simulink model "gm_TapFilter"  (R2017a)
settings: Solver=VariableStepAuto  StartTime=0.0  StopTime=10.0  RelTol=1e-3
settings Model: Creator=Arthur  LastModifiedBy=Arthur
settings OptimizationCC: BlockReduction=off  ConditionallyExecuteInputs=off
settings DebuggingCC: InheritedTsInSrcMsg=none

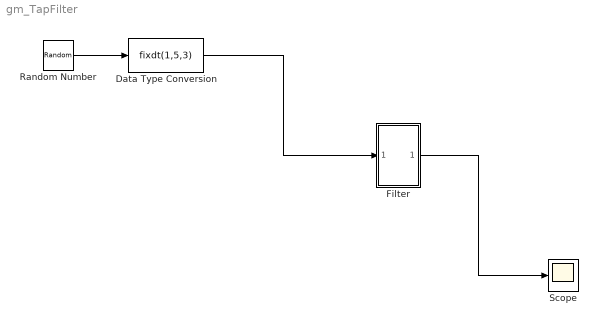
== system gm_TapFilter ==
  Data Type Conversion : DataTypeConversion  OutDataTypeStr=fixdt(1,5,3)
  Filter : Subsystem
  Random Number : RandomNumber  SampleTime=0.1
  Scope : Scope
  wires:
  Filter/1(Out1) -> Scope/1
  Data Type Conversion/1 -> Filter/1(In1)
  Random Number/1 -> Data Type Conversion/1

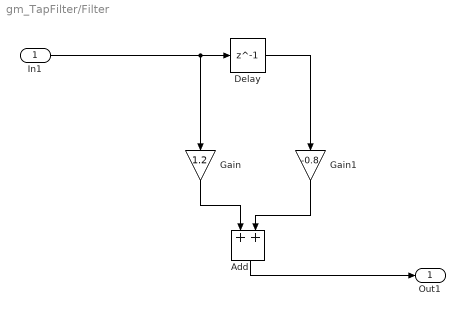
== system gm_TapFilter/Filter ==
  In1 : Inport
  Add : Sum  OutDataTypeStr=fixdt(1,5,2)
  Delay : Delay  DelayLength=1
  Gain : Gain  Gain=1.2  ParamDataTypeStr=fixdt(1,5,3)  OutDataTypeStr=fixdt(1,6,3)
  Gain1 : Gain  Gain=-0.8  ParamDataTypeStr=fixdt(1,6,3)  OutDataTypeStr=fixdt(1,5,3)
  Out1 : Outport
  wires:
  Delay/1 -> Gain1/1
  Gain1/1 -> Add/2
  Gain/1 -> Add/1
  In1/1 -> Delay/1, Gain/1
  Add/1 -> Out1/1
